simulink model "suspenauto"  (R2022b)
settings: Solver=VariableStepAuto  StartTime=0.0  StopTime=10.0  RelTol=1e-3
values from neighbouring files (symbols this model uses):
  b1 = 1000    [autosuspara.m]    (also in cuartosuspenauto.m)
  f = 0    [autosuspara.m]    (also in cuartosuspenauto.m)
  k1 = 16182    [autosuspara.m]    (also in cuartosuspenauto.m)
  k2 = 19000    [autosuspara.m]    (also in cuartosuspenauto.m)
  m1 = 290    [autosuspara.m]    (also in cuartosuspenauto.m)
  m2 = 59    [autosuspara.m]    (also in cuartosuspenauto.m)
libraries: fl_lib x11, nesl_utility x4
settings Model: Creator=mluser  LastModifiedBy=mluser

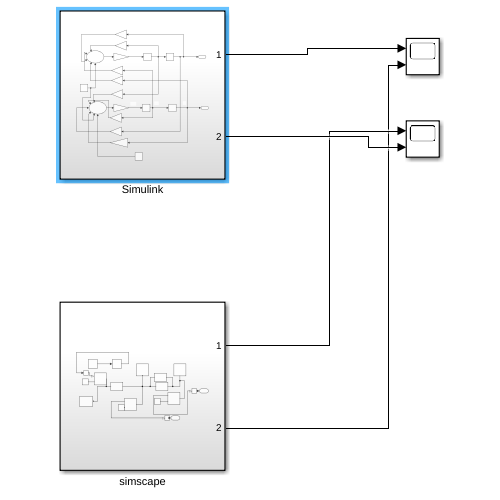
[thumbnail: Simulink's stored preview of the top-level diagram]
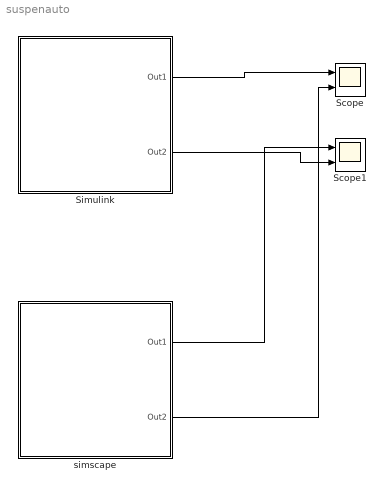
== system suspenauto ==
  Scope : Scope  NumInputPorts=2
  Scope1 : Scope  NumInputPorts=2
  Simulink : Subsystem
  simscape : Subsystem
  wires:
  Simulink/1(Out1) -> Scope/1
  Simulink/2(Out2) -> Scope1/2
  simscape/1(Out1) -> Scope1/1
  simscape/2(Out2) -> Scope/2

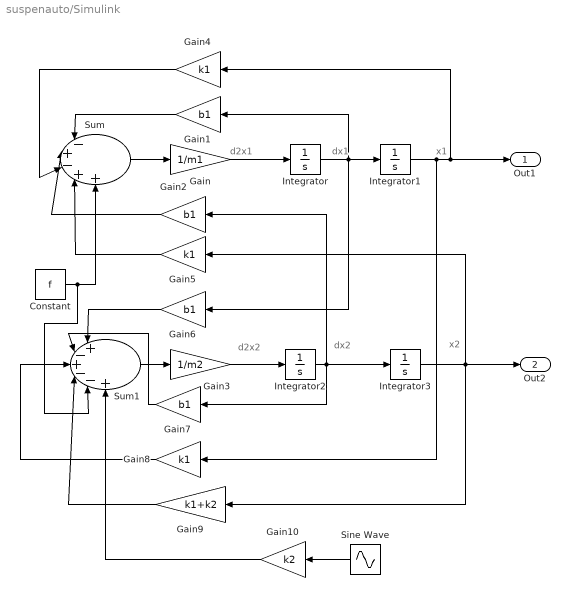
== system suspenauto/Simulink ==
  note: d2x1
  note: dx1
  note: x1
  note: x2
  note: d2x2
  note: dx2
  Constant : Constant  Value=f
  Gain : Gain  Gain=1/m1
  Gain{1..2,6..7} (4 alike) : Gain  Gain=b1
  Gain10 : Gain  Gain=k2
  Gain3 : Gain  Gain=1/m2
  Gain4 : Gain  Gain=k1
  Gain5 : Gain  Gain=k1
  Gain8 : Gain  Gain=k1
  Gain9 : Gain  Gain=k1+k2
  Integrator{,1..3} (4 alike) : Integrator
  Sine Wave : Sin  Amplitude=0.05  Frequency=0.5*pi  SampleTime=0
  Sum : Sum  Inputs=|-+-++
  Sum1 : Sum  Inputs=|+-+--+
  Out1 : Outport
  Out2 : Outport  Port=2
  wires:
  Gain1/1 -> Sum/1
  Integrator1/1 -> Gain4/1, Out1/1, Gain8/1
  Integrator3/1 -> Gain9/1, Gain5/1, Out2/1
  Sum/1 -> Gain/1
  Integrator2/1 -> Gain7/1, Integrator3/1, Gain2/1
  Gain3/1 -> Integrator2/1
  Sum1/1 -> Gain3/1
  Gain/1 -> Integrator/1
  Integrator/1 -> Gain6/1, Gain1/1, Integrator1/1
  Gain2/1 -> Sum/2
  Gain4/1 -> Sum/3
  Gain5/1 -> Sum/4
  Constant/1 -> Sum1/5, Sum/5
  Gain6/1 -> Sum1/1
  Gain7/1 -> Sum1/2
  Gain8/1 -> Sum1/3
  Gain9/1 -> Sum1/4
  Gain10/1 -> Sum1/6
  Sine Wave/1 -> Gain10/1

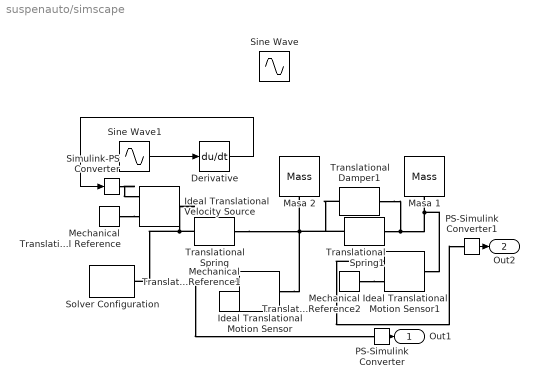
== system suspenauto/simscape ==
  Derivative : Derivative
  Ideal Translational Motion Sensor : fl_lib/Mechanical/Mechanical Sensors/Ideal Translational Motion Sensor  reference=foundation.enum.MeasurementReference.difference  acceleration_port=false  velocity_port=false  position_port=true  offset=0 m
      settings: InternalSimscapePortConfiguration="{\"Bottom\":[],\"Left\":[{\"id\":\"R\",\"label\":\"R\",\"type\":\"foundation.mechanical.translational.translational\"}],\"Right\":[{\"id\":\"C\",\"label\":\"C\",\"type\":\"foundation.mechanical.translational.translational\"},{\"id\":\"P\",\"label\":\"P\",\"type\":\"output\"}],\"Top\":[]}"
  Ideal Translational Motion Sensor1 : fl_lib/Mechanical/Mechanical Sensors/Ideal Translational Motion Sensor  reference=foundation.enum.MeasurementReference.difference  acceleration_port=false  velocity_port=false  position_port=true  offset=0 m
      settings: InternalSimscapePortConfiguration="{\"Bottom\":[],\"Left\":[{\"id\":\"R\",\"label\":\"R\",\"type\":\"foundation.mechanical.translational.translational\"}],\"Right\":[{\"id\":\"C\",\"label\":\"C\",\"type\":\"foundation.mechanical.translational.translational\"},{\"id\":\"P\",\"label\":\"P\",\"type\":\"output\"}],\"Top\":[]}"
  Ideal Translational Velocity Source : fl_lib/Mechanical/Mechanical Sources/Ideal Translational Velocity Source
  Masa 1 : fl_lib/Mechanical/Translational Elements/Mass  mass=290 kg  num_ports=foundation.enum.numPorts2.one  v_specify=off  v_priority=High  v=0.05*sin(0.5*pi) m/s  v_nominal_specify=off  v_nominal_unit=m/s  v_nominal_value=1  f_specify=off  f_priority=None  f=0 N  f_nominal_specify=off  f_nominal_unit=N  f_nominal_value=1
  "Masa 2 " : fl_lib/Mechanical/Translational Elements/Mass  mass=59 kg  num_ports=foundation.enum.numPorts2.one  v_specify=off  v_priority=High  v=0.05*sin(0.5*pi) m/s  v_nominal_specify=off  v_nominal_unit=m/s  v_nominal_value=1  f_specify=off  f_priority=None  f=0 N  f_nominal_specify=off  f_nominal_unit=N  f_nominal_value=1
  Mechanical Translational Reference : fl_lib/Mechanical/Translational Elements/Mechanical Translational Reference
  Mechanical Translational Reference1 : fl_lib/Mechanical/Translational Elements/Mechanical Translational Reference
  Mechanical Translational Reference2 : fl_lib/Mechanical/Translational Elements/Mechanical Translational Reference
  PS-Simulink Converter : nesl_utility/PS-Simulink Converter  PhysicalDomain=network_engine_domain  SubClassName=ps_output  LeftPortType=input  RightPortType=output  PseudoPeriodic=off  Frequencies=[]  VectorFormat=inherit  Unit=inherit  AffineConversion=off
  PS-Simulink Converter1 : nesl_utility/PS-Simulink Converter  PhysicalDomain=network_engine_domain  SubClassName=ps_output  LeftPortType=input  RightPortType=output  PseudoPeriodic=off  Frequencies=[]  VectorFormat=inherit  Unit=inherit  AffineConversion=off
  Simulink-PS Converter : nesl_utility/Simulink-PS Converter  PhysicalDomain=network_engine_domain  SubClassName=ps_input  LeftPortType=input  RightPortType=output  PseudoPeriodic=off  Frequencies=[]  NoiseDistribution=none  NoiseParameters=[]  Unit=1  AffineConversion=off  FilteringAndDerivatives=provide  SimscapeFilterOrder=1  InputFilterTimeConstant=0.001  UdotUserProvided=0
  Sine Wave : Sin  Amplitude=0.05  Frequency=0.5*pi  SampleTime=0
  Sine Wave1 : Sin  Amplitude=0.05  Frequency=0.5*pi  SampleTime=0
  Solver Configuration : nesl_utility/Solver Configuration  PhysicalDomain=network_engine_domain  SubClassName=solver  LeftPortType=input  RightPortType=generic  Tones=[]  Harmonics=[]  SimulateNoise=off  Profile=off  UseLocalSampling=off  EnableSwitchedLinearOptims=on  FrequencyDomain=off  UseCCode=off  RelTol=0.001  AbsTol=0.001  MinStep=1e-09  ToWorkspace=off  RevertToSquareIcSolve=off  NumHomotopyIterations=100  PhasorMode=off  PhasorModeNumHarmonics=1  ConsistencySolver=NEWTON_XTOL_AFTER_FTOL  IndexReductionMethod=DerivativeReplacement  DoDC=off  ResidualTolerance=1e-09  ConsistencyTolSource=GLOBAL  ConsistencyAbsTol=0.001  ConsistencyRelTol=0.001  ConsistencyTolFactor=0.001  UseLocalSolver=off  LocalSolverChoice=NE_BACKWARD_EULER_ADVANCER  ResolveIndetEquations=on  FunctionEvalNumThread=1  LocalSolverSampleTime=0.001  DoFixedCost=off  MaxNonlinIter=3  MaxModeIter=2  ComputeImpulses=off  ImpulseIterations=2  LinearAlgebra=auto  LinearAlgebraNumThread=0  EquationFormulation=NE_TIME_EF  DelaysMemoryBudget=1024  AutomaticFiltering=on  FilteringTimeConstant=0.001  PartitionStorageMethod=AS_NEEDED  PartitionMemoryBudget=1024  PartitionMethod=ROBUST
  Translational Damper1 : fl_lib/Mechanical/Translational Elements/Translational Damper  D=1000 N*s/m  v_specify=off  v_priority=None  v=0 m/s  v_nominal_specify=off  v_nominal_unit=m/s  v_nominal_value=1  f_specify=off  f_priority=None  f=0 N  f_nominal_specify=off  f_nominal_unit=N  f_nominal_value=1
  Translational Spring : fl_lib/Mechanical/Translational Elements/Translational Spring  spr_rate=19000 N/m  v_specify=off  v_priority=None  v=0.05*sin(0.5*pi) m/s  v_nominal_specify=off  v_nominal_unit=m/s  v_nominal_value=1  f_specify=off  f_priority=None  f=0 N  f_nominal_specify=off  f_nominal_unit=N  f_nominal_value=1  x_specify=off  x_priority=High  x=0.05*sin(0.5*pi) m  x_nominal_specify=off  x_nominal_unit=m  x_nominal_value=0.05*sin(0.5*pi)
  Translational Spring1 : fl_lib/Mechanical/Translational Elements/Translational Spring  spr_rate=16182 N/m  v_specify=off  v_priority=None  v=0.05 m/s  v_nominal_specify=off  v_nominal_unit=m/s  v_nominal_value=1  f_specify=off  f_priority=None  f=0 N  f_nominal_specify=off  f_nominal_unit=N  f_nominal_value=1  x_specify=off  x_priority=High  x=0.05*sin(0.5*pi) m  x_nominal_specify=off  x_nominal_unit=m  x_nominal_value=1
  Out1 : Outport
  Out2 : Outport  Port=2
  wires:
  PS-Simulink Converter/1 -> Out1/1
  PS-Simulink Converter1/1 -> Out2/1
  Sine Wave1/1 -> Derivative/1
  Derivative/1 -> Simulink-PS Converter/1
  connections:
  Translational Spring/LConn1 -- Solver Configuration/RConn1 -- Ideal Translational Velocity Source/LConn1
  Translational Spring/RConn1 -- Translational Damper1/LConn1 -- Translational Spring1/LConn1 -- Ideal Translational Motion Sensor/LConn1 -- "Masa 2 "/LConn1
  Translational Spring1/RConn1 -- Translational Damper1/RConn1 -- Ideal Translational Motion Sensor1/LConn1 -- Masa 1/LConn1
  Mechanical Translational Reference1/LConn1 -- Ideal Translational Motion Sensor/RConn1
  Ideal Translational Motion Sensor/RConn2 -- PS-Simulink Converter/LConn1
  Ideal Translational Motion Sensor1/RConn2 -- PS-Simulink Converter1/LConn1
  Mechanical Translational Reference2/LConn1 -- Ideal Translational Motion Sensor1/RConn1
  Mechanical Translational Reference/LConn1 -- Ideal Translational Velocity Source/RConn2
  Simulink-PS Converter/RConn1 -- Ideal Translational Velocity Source/RConn1
